simulink model "CRIntegrator"  (Simulink 6.6)
settings: Solver=FixedStepDiscrete  SolverMode=SingleTasking  StartTime=0.0  StopTime=50  FixedStep=sample  RelTol=1e-3
values from neighbouring files (symbols this model uses):
  Keq = 3.92e6*1    (= 3920000)    [Alpha_init_setup.m]
  steps = length(p1)    [Alpha_init_setup.m]
undefined symbols (not defined in the file or in its folder): beta1, beta2, C, Ceq, dt, dt_multiplier, K, Minv, sample
settings Model: Creator=Tommy  LastModifiedBy=Tommy  BufferReuse=off
settings OptimizationCC: BlockReduction=off  OptimizeBlockIOStorage=off  BufferReuse=off  ExpressionFolding=off  LocalBlockOutputs=off
settings DebuggingCC: MultiTaskCondExecSysMsg=none
settings RTWCC: SystemTargetFile=xpctarget.tlc  TemplateMakefile=xpc_default_tmf  Description=xPC Target  ProcessScript=xpctarget_make_rtw_hook  IncludeERTFirstTime=on
settings xpcTargetCC: TargetFcnLib=ansi_tfl_tmw.mat  GenFloatMathFcnCalls=ANSI_C  PortableWordSizes=off

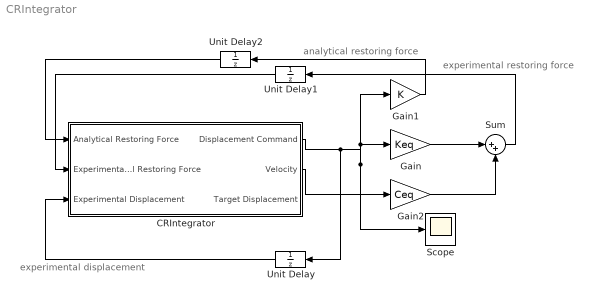
== system CRIntegrator ==
  note: experimental restoring force
  note: analytical restoring force
  note: experimental displacement
  CRIntegrator : Subsystem
  Gain : Gain  Gain=Keq  SampleTime=sample
  Gain1 : Gain  Gain=K  SampleTime=sample
  Gain2 : Gain  Gain=Ceq  SampleTime=sample
  Scope : Scope
      settings: TimeRange=50  YMin=-0.01  YMax=0.01  MaxDataPoints=50000000
  Sum : Sum  Inputs=|++  SampleTime=sample
  Unit Delay : UnitDelay  Orientation=left  SampleTime=sample
  Unit Delay1 : UnitDelay  Orientation=left  SampleTime=sample
  Unit Delay2 : UnitDelay  Orientation=left  SampleTime=sample
  wires:
  CRIntegrator/1(Displacement Command) -> Gain/1, Gain1/1, Scope/1, Unit Delay/1
  CRIntegrator/2(Velocity) -> Gain2/1
  Gain2/1 -> Sum/2
  Gain/1 -> Sum/1
  Sum/1 -> Unit Delay1/1
  Gain1/1 -> Unit Delay2/1
  Unit Delay/1 -> CRIntegrator/3(Experimental Displacement)
  Unit Delay1/1 -> CRIntegrator/2(Experimental Restoring Force)
  Unit Delay2/1 -> CRIntegrator/1(Analytical Restoring Force)

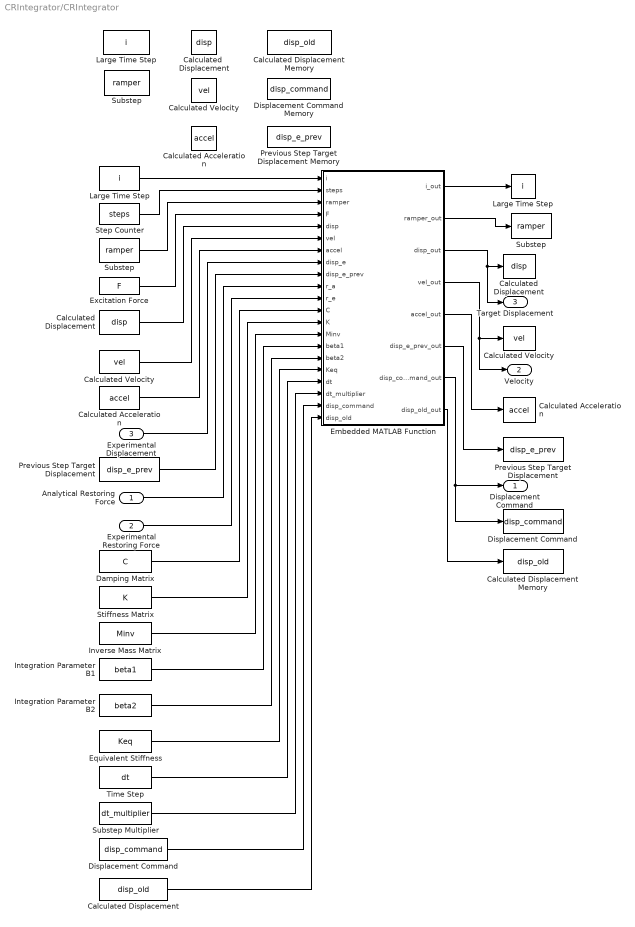
== system CRIntegrator/CRIntegrator ==
  Analytical Restoring Force : Inport
  Experimental Restoring Force : Inport  Port=2
  Experimental Displacement : Inport  Port=3
  " Calculated Acceleration" : DataStoreWrite  DataStoreName=accel  SampleTime=sample
  " Calculated Displacement" : DataStoreWrite  DataStoreName=disp  SampleTime=sample
  " Calculated Displacement Memory" : DataStoreWrite  DataStoreName=disp_old  SampleTime=sample
  " Calculated Velocity" : DataStoreWrite  DataStoreName=vel  SampleTime=sample
  " Displacement Command" : DataStoreWrite  DataStoreName=disp_command  SampleTime=sample
  " Large Time Step" : DataStoreWrite  DataStoreName=i  SampleTime=sample
  " Previous Step Target Displacement" : DataStoreWrite  DataStoreName=disp_e_prev  SampleTime=sample
  " Substep" : DataStoreWrite  DataStoreName=ramper  SampleTime=sample
  Calculated Acceleration : DataStoreMemory  DataStoreName=accel  InitialValue=0
  Calculated Velocity : DataStoreMemory  DataStoreName=vel  InitialValue=0
  Calculated  Displacement : DataStoreMemory  DataStoreName=disp  InitialValue=0
  "Calculated Acceleration " : DataStoreRead  DataStoreName=accel  SampleTime=sample
  Calculated Displacement : DataStoreRead  DataStoreName=disp_old  SampleTime=sample
  Calculated Displacement Memory : DataStoreMemory  DataStoreName=disp_old  InitialValue=0
  "Calculated Displacement " : DataStoreRead  DataStoreName=disp  SampleTime=sample
  "Calculated Velocity " : DataStoreRead  DataStoreName=vel  SampleTime=sample
  Damping Matrix : Constant  Value=C  SampleTime=sample
  Displacement Command Memory : DataStoreMemory  DataStoreName=disp_command  InitialValue=0
  "Displacement Command " : DataStoreRead  DataStoreName=disp_command  SampleTime=sample
  Embedded MATLAB Function : Stateflow chart
  Equivalent Stiffness : Constant  Value=Keq  SampleTime=sample
  Excitation Force : FromWorkspace  VariableName=F  SampleTime=0
  Integration Parameter B1 : Constant  Value=beta1  SampleTime=sample
  Integration Parameter B2 : Constant  Value=beta2  SampleTime=sample
  Inverse Mass Matrix : Constant  Value=Minv  SampleTime=sample
  Large Time Step : DataStoreMemory  DataStoreName=i  InitialValue=0
  "Large Time Step " : DataStoreRead  DataStoreName=i  SampleTime=sample
  Previous Step Target Displacement Memory : DataStoreMemory  DataStoreName=disp_e_prev  InitialValue=0
  Previous Step Target Displacement : DataStoreRead  DataStoreName=disp_e_prev  SampleTime=sample
  Step Counter : Constant  Value=steps  SampleTime=sample
  Stiffness Matrix : Constant  Value=K  SampleTime=sample
  Substep : DataStoreMemory  DataStoreName=ramper  InitialValue=1
  "Substep " : DataStoreRead  DataStoreName=ramper  SampleTime=sample
  Substep Multiplier : Constant  Value=dt_multiplier  SampleTime=sample
  Time Step : Constant  Value=dt  SampleTime=sample
  Displacement Command : Outport
  Velocity : Outport  Port=2
  Target Displacement : Outport  Port=3
  wires:
  "Large Time Step "/1 -> Embedded MATLAB Function/1(i)
  Excitation Force/1 -> Embedded MATLAB Function/4(F)
  Damping Matrix/1 -> Embedded MATLAB Function/12(C)
  Stiffness Matrix/1 -> Embedded MATLAB Function/13(K)
  Inverse Mass Matrix/1 -> Embedded MATLAB Function/14(Minv)
  Substep Multiplier/1 -> Embedded MATLAB Function/19(dt_multiplier)
  Embedded MATLAB Function/4(vel_out) -> Velocity/1, " Calculated Velocity"/1
  Embedded MATLAB Function/7(disp_command_out) -> Displacement Command/1, " Displacement Command"/1
  Analytical Restoring Force/1 -> Embedded MATLAB Function/10(r_a)
  Experimental Restoring Force/1 -> Embedded MATLAB Function/11(r_e)
  Experimental Displacement/1 -> Embedded MATLAB Function/8(disp_e)
  Time Step/1 -> Embedded MATLAB Function/18(dt)
  Equivalent Stiffness/1 -> Embedded MATLAB Function/17(Keq)
  Step Counter/1 -> Embedded MATLAB Function/2(steps)
  Integration Parameter B1/1 -> Embedded MATLAB Function/15(beta1)
  Integration Parameter B2/1 -> Embedded MATLAB Function/16(beta2)
  Embedded MATLAB Function/1(i_out) -> " Large Time Step"/1
  Embedded MATLAB Function/2(ramper_out) -> " Substep"/1
  Embedded MATLAB Function/3(disp_out) -> " Calculated Displacement"/1, Target Displacement/1
  Embedded MATLAB Function/5(accel_out) -> " Calculated Acceleration"/1
  Embedded MATLAB Function/6(disp_e_prev_out) -> " Previous Step Target Displacement"/1
  Embedded MATLAB Function/8(disp_old_out) -> " Calculated Displacement Memory"/1
  "Substep "/1 -> Embedded MATLAB Function/3(ramper)
  "Calculated Displacement "/1 -> Embedded MATLAB Function/5(disp)
  "Calculated Velocity "/1 -> Embedded MATLAB Function/6(vel)
  "Calculated Acceleration "/1 -> Embedded MATLAB Function/7(accel)
  Previous Step Target Displacement/1 -> Embedded MATLAB Function/9(disp_e_prev)
  "Displacement Command "/1 -> Embedded MATLAB Function/20(disp_command)
  Calculated Displacement/1 -> Embedded MATLAB Function/21(disp_old)

== matlab function CRIntegrator/Embedded MATLAB Function ==
  data: i input inherited; steps input inherited; i_out output inherited; ramper_out output inherited; ramper input inherited; F input inherited; disp input inherited; vel input inherited; accel input inherited; disp_e input inherited; disp_e_prev input inherited; r_a input inherited; r_e input inherited; C input inherited; K input inherited; Minv input inherited; disp_out output inherited; vel_out output inherited; accel_out output inherited; disp_e_prev_out output inherited; beta1 input inherited; beta2 input inherited; Keq input inherited; dt input inherited; dt_multiplier input inherited; disp_command input inherited; disp_command_out output inherited; disp_old_out output inherited; disp_old input inherited
function [i_out,ramper_out,disp_out,vel_out,accel_out,disp_e_prev_out,disp_command_out,disp_old_out]  = fcn(i,steps,ramper,F,disp,vel,accel,disp_e,disp_e_prev,r_a,r_e,C,K,Minv,beta1,beta2,Keq,dt,dt_multiplier,disp_command,disp_old)
 
%% First step initializes acceleration vector
if (i == 0)
    accel = Minv*( F(1)-C*vel-K*disp ); %calculate new acceleration vector
end

%% Main cycle occurs while the earthquake record isn't exhausted
if (i < steps-1)  
    %% First ramp of a new step, calculate displacement and velocity vectors
    if (ramper == 1)
        i = i + 1;                                  %increment to next step
        disp_old = disp;                            %save previous displacement
        disp = disp + dt*vel + beta2*dt^2*accel;    %calculate next displacement vector
        vel = vel + beta1*dt*accel;                 %calculate next velocity vector
        disp_e_prev = disp_e;                       %get initial displacement for this step      
    end
    
    %% Set ramped command vector
    disp_command_out = (disp - disp_old)/dt_multiplier * ramper + disp_old;
    
    %% Check for the last ramper
    if (ramper == dt_multiplier)
        ramper_out = 1;      
        r_e = r_e + Keq*(disp_e - disp_e_prev)/dt_multiplier;  %correct restoring force                
        r = r_e + r_a;                   %form full restoring force vector                
        accel = Minv*( F(i)-C*vel-r ); %calculate new acceleration vector
    %% Ramp the command within the same earthquake step
    else
        ramper_out = ramper + 1;
    end
    
    %% Pass variables through to the next sample 
    i_out = i;                  %remember big time step
    disp_out = disp;            %remember displacement vector
    vel_out = vel;              %remember velocity vector
    accel_out = accel;          %remember acceleration vector
    disp_old_out = disp_old;    %remember previous displacement vector
    disp_e_prev_out = disp_e_prev; %remember initial measured experimental displacement
          
%% Earthquake record exhausted so just set output = input for all variables
else
    i_out = i;
    ramper_out = ramper;
    disp_out = disp;    
    vel_out = vel;      
    accel_out = accel;
    disp_command_out = disp_command; 
    disp_old_out = disp_old;
    disp_e_prev_out = disp_e_prev;
end
